simulink model "sistemaPID"  (R2024b)
settings: Solver=VariableStepAuto  StartTime=0.0  StopTime=10.0  RelTol=1e-3
settings Model: Creator=estel  LastModifiedBy=estel

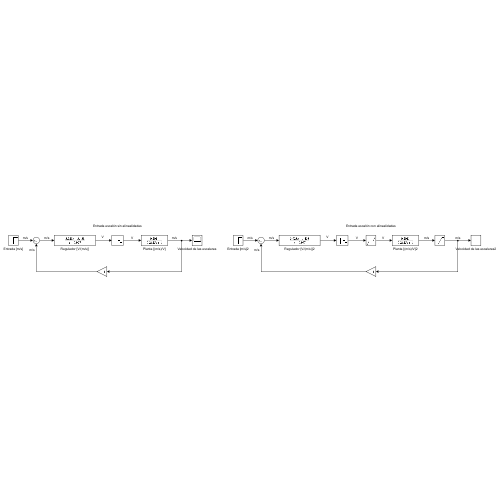
[thumbnail: Simulink's stored preview of the top-level diagram]
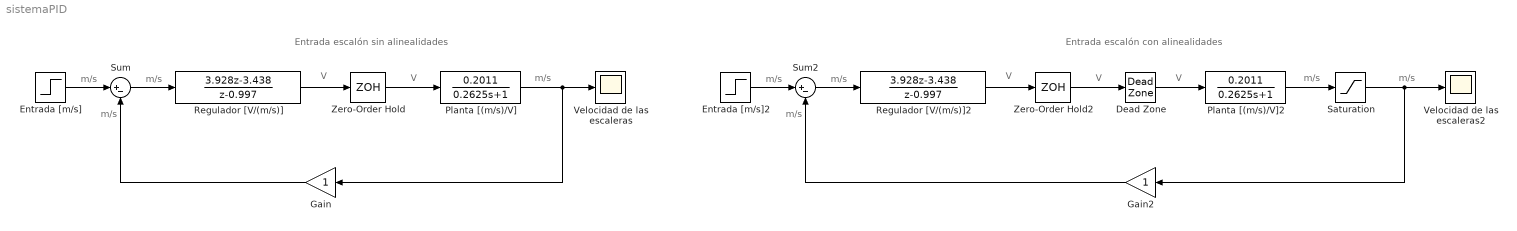
== system sistemaPID ==
  note: Entrada escalón sin alinealidades
  note: m/s
  note: m/s
  note: m/s
  note: m/s
  note: V
  note: V
  note: Entrada escalón con alinealidades
  note: m/s
  note: m/s
  note: m/s
  note: m/s
  note: V
  note: V
  note: m/s
  note: V
  Dead Zone : DeadZone  LowerValue=-0.19  UpperValue=0.19
  Entrada [m/s] : Step  SampleTime=0
  Entrada [m/s]2 : Step  SampleTime=0
  Gain : Gain
  Gain2 : Gain
  Planta [(m/s)/V] : TransferFcn  Numerator=[0.2011]  Denominator=[0.2625 1]
  Planta [(m/s)/V]2 : TransferFcn  Numerator=[0.2011]  Denominator=[0.2625 1]
  Regulador [V/(m/s)] : DiscreteTransferFcn  Numerator=[3.928 -3.438]  Denominator=[1 -0.997]
  Regulador [V/(m/s)]2 : DiscreteTransferFcn  Numerator=[3.928 -3.438]  Denominator=[1 -0.997]
  Saturation : Saturate  UpperLimit=10  LowerLimit=-10
  Sum : Sum  Inputs=|+-
  Sum2 : Sum  Inputs=|+-
  Velocidad de las escaleras : Scope
  Velocidad de las escaleras2 : Scope
  Zero-Order Hold : ZeroOrderHold  SampleTime=-1
  Zero-Order Hold2 : ZeroOrderHold  SampleTime=-1
  wires:
  Entrada [m/s]/1 -> Sum/1
  Sum/1 -> Regulador [V/(m/s)]/1
  Regulador [V/(m/s)]/1 -> Zero-Order Hold/1
  Zero-Order Hold/1 -> Planta [(m/s)/V]/1
  Planta [(m/s)/V]/1 -> Gain/1, Velocidad de las escaleras/1
  Gain/1 -> Sum/2
  Gain2/1 -> Sum2/2
  Regulador [V/(m/s)]2/1 -> Zero-Order Hold2/1
  Sum2/1 -> Regulador [V/(m/s)]2/1
  Entrada [m/s]2/1 -> Sum2/1
  Planta [(m/s)/V]2/1 -> Saturation/1
  Saturation/1 -> Gain2/1, Velocidad de las escaleras2/1
  Dead Zone/1 -> Planta [(m/s)/V]2/1
  Zero-Order Hold2/1 -> Dead Zone/1
